simulink model "fusionAlg"  (R2018b)
settings: Solver=FixedStepDiscrete  StartTime=0.0  StopTime=inf  FixedStep=0.01  RelTol=1e-3
PostLoadFcn:
  | if any(exist('dsrtsu_mdlpostloadfcn', 'file') ~= 0), dsrtsu_mdlpostloadfcn('Execute', bdroot); end
model workspace (MAT data in the model file):
  handle : class17 (value not decoded)
(part 13 of 24)

== system fusionAlg/FUSION /FUS_DataAdapter/ARS308Adapter/leftFrontRadar/Subsystem1/OBJ_20 ==
  OBJ_01 : Inport
  Bus Creator : BusCreator  Inputs=2  OutDataTypeStr=Bus: FUS_UINT8_RESERVED_ST
      settings: InheritFromInputs=off
  Bus Creator1 : BusCreator  Inputs=17  OutDataTypeStr=Bus: FUS_RADAR_OBJ_ST  NonVirtualBus=on
      settings: InheritFromInputs=off
  Bus Selector1 : BusSelector  OutputSignals=RCS,VrelLat,VrelLong,DistLong,DistLat,ID,DynProp
  Constant{,1,8..10} (5 alike) : Constant  Value=0  OutDataTypeStr=uint8
  Constant{2..6} (5 alike) : Constant  Value=0  OutDataTypeStr=single
  Constant7 : Constant  OutDataTypeStr=uint8
  Data Type Conversion : DataTypeConversion  OutDataTypeStr=uint16
  Data Type Conversion1 : DataTypeConversion  OutDataTypeStr=uint8
  Switch : Switch  Criteria=u2 > Threshold  OutDataTypeStr=uint8
  <OBJ_01> : Outport
  wires:
  Constant1/1 -> Bus Creator/2
  Bus Creator1/1 -> <OBJ_01>/1
  Constant/1 -> Bus Creator/1
  OBJ_01/1 -> Bus Selector1/1
  Bus Creator/1 -> Bus Creator1/17
  Bus Selector1/1 -> Bus Creator1/1  "<RCS>"
  Constant2/1 -> Bus Creator1/2  "XPos_STD"
  Constant3/1 -> Bus Creator1/3  "YPos_STD"
  Constant4/1 -> Bus Creator1/4  "XVelRel_STD"
  Constant5/1 -> Bus Creator1/5  "XAccRel"
  Constant6/1 -> Bus Creator1/6  "ExstProb"
  Bus Selector1/2 -> Bus Creator1/7  "<VrelLat>"
  Bus Selector1/3 -> Bus Creator1/8  "<VrelLong>"
  Bus Selector1/4 -> Bus Creator1/9  "<DistLong>"
  Bus Selector1/5 -> Bus Creator1/10  "<DistLat>"
  Bus Selector1/6 -> Data Type Conversion/1  "<ID>"
  Data Type Conversion/1 -> Bus Creator1/11, Switch/2
  Constant8/1 -> Switch/3  "ValidFlag"
  Bus Selector1/7 -> Data Type Conversion1/1  "<DynProp>"
  Constant9/1 -> Bus Creator1/15  "Type"
  Constant10/1 -> Bus Creator1/16  "MeasFlag"
  Data Type Conversion1/1 -> Bus Creator1/14
  Constant7/1 -> Switch/1  "UpdateFlag"
  Switch/1 -> Bus Creator1/13, Bus Creator1/12

== system fusionAlg/FUSION /FUS_DataAdapter/ARS308Adapter/leftFrontRadar/Subsystem1/OBJ_21 ==
  OBJ_01 : Inport
  Bus Creator : BusCreator  Inputs=2  OutDataTypeStr=Bus: FUS_UINT8_RESERVED_ST
      settings: InheritFromInputs=off
  Bus Creator1 : BusCreator  Inputs=17  OutDataTypeStr=Bus: FUS_RADAR_OBJ_ST  NonVirtualBus=on
      settings: InheritFromInputs=off
  Bus Selector1 : BusSelector  OutputSignals=RCS,VrelLat,VrelLong,DistLong,DistLat,ID,DynProp
  Constant{,1,8..10} (5 alike) : Constant  Value=0  OutDataTypeStr=uint8
  Constant{2..6} (5 alike) : Constant  Value=0  OutDataTypeStr=single
  Constant7 : Constant  OutDataTypeStr=uint8
  Data Type Conversion : DataTypeConversion  OutDataTypeStr=uint16
  Data Type Conversion1 : DataTypeConversion  OutDataTypeStr=uint8
  Switch : Switch  Criteria=u2 > Threshold  OutDataTypeStr=uint8
  <OBJ_01> : Outport
  wires:
  Constant1/1 -> Bus Creator/2
  Bus Creator1/1 -> <OBJ_01>/1
  Constant/1 -> Bus Creator/1
  OBJ_01/1 -> Bus Selector1/1
  Bus Creator/1 -> Bus Creator1/17
  Bus Selector1/1 -> Bus Creator1/1  "<RCS>"
  Constant2/1 -> Bus Creator1/2  "XPos_STD"
  Constant3/1 -> Bus Creator1/3  "YPos_STD"
  Constant4/1 -> Bus Creator1/4  "XVelRel_STD"
  Constant5/1 -> Bus Creator1/5  "XAccRel"
  Constant6/1 -> Bus Creator1/6  "ExstProb"
  Bus Selector1/2 -> Bus Creator1/7  "<VrelLat>"
  Bus Selector1/3 -> Bus Creator1/8  "<VrelLong>"
  Bus Selector1/4 -> Bus Creator1/9  "<DistLong>"
  Bus Selector1/5 -> Bus Creator1/10  "<DistLat>"
  Bus Selector1/6 -> Data Type Conversion/1  "<ID>"
  Data Type Conversion/1 -> Bus Creator1/11, Switch/2
  Constant8/1 -> Switch/3  "ValidFlag"
  Bus Selector1/7 -> Data Type Conversion1/1  "<DynProp>"
  Constant9/1 -> Bus Creator1/15  "Type"
  Constant10/1 -> Bus Creator1/16  "MeasFlag"
  Data Type Conversion1/1 -> Bus Creator1/14
  Constant7/1 -> Switch/1  "UpdateFlag"
  Switch/1 -> Bus Creator1/13, Bus Creator1/12

== system fusionAlg/FUSION /FUS_DataAdapter/ARS308Adapter/leftFrontRadar/Subsystem1/OBJ_22 ==
  OBJ_01 : Inport
  Bus Creator : BusCreator  Inputs=2  OutDataTypeStr=Bus: FUS_UINT8_RESERVED_ST
      settings: InheritFromInputs=off
  Bus Creator1 : BusCreator  Inputs=17  OutDataTypeStr=Bus: FUS_RADAR_OBJ_ST  NonVirtualBus=on
      settings: InheritFromInputs=off
  Bus Selector1 : BusSelector  OutputSignals=RCS,VrelLat,VrelLong,DistLong,DistLat,ID,DynProp
  Constant{,1,8..10} (5 alike) : Constant  Value=0  OutDataTypeStr=uint8
  Constant{2..6} (5 alike) : Constant  Value=0  OutDataTypeStr=single
  Constant7 : Constant  OutDataTypeStr=uint8
  Data Type Conversion : DataTypeConversion  OutDataTypeStr=uint16
  Data Type Conversion1 : DataTypeConversion  OutDataTypeStr=uint8
  Switch : Switch  Criteria=u2 > Threshold  OutDataTypeStr=uint8
  <OBJ_01> : Outport
  wires:
  Constant1/1 -> Bus Creator/2
  Bus Creator1/1 -> <OBJ_01>/1
  Constant/1 -> Bus Creator/1
  OBJ_01/1 -> Bus Selector1/1
  Bus Creator/1 -> Bus Creator1/17
  Bus Selector1/1 -> Bus Creator1/1  "<RCS>"
  Constant2/1 -> Bus Creator1/2  "XPos_STD"
  Constant3/1 -> Bus Creator1/3  "YPos_STD"
  Constant4/1 -> Bus Creator1/4  "XVelRel_STD"
  Constant5/1 -> Bus Creator1/5  "XAccRel"
  Constant6/1 -> Bus Creator1/6  "ExstProb"
  Bus Selector1/2 -> Bus Creator1/7  "<VrelLat>"
  Bus Selector1/3 -> Bus Creator1/8  "<VrelLong>"
  Bus Selector1/4 -> Bus Creator1/9  "<DistLong>"
  Bus Selector1/5 -> Bus Creator1/10  "<DistLat>"
  Bus Selector1/6 -> Data Type Conversion/1  "<ID>"
  Data Type Conversion/1 -> Bus Creator1/11, Switch/2
  Constant8/1 -> Switch/3  "ValidFlag"
  Bus Selector1/7 -> Data Type Conversion1/1  "<DynProp>"
  Constant9/1 -> Bus Creator1/15  "Type"
  Constant10/1 -> Bus Creator1/16  "MeasFlag"
  Data Type Conversion1/1 -> Bus Creator1/14
  Constant7/1 -> Switch/1  "UpdateFlag"
  Switch/1 -> Bus Creator1/13, Bus Creator1/12

== system fusionAlg/FUSION /FUS_DataAdapter/ARS308Adapter/leftFrontRadar/Subsystem1/OBJ_23 ==
  OBJ_01 : Inport
  Bus Creator : BusCreator  Inputs=2  OutDataTypeStr=Bus: FUS_UINT8_RESERVED_ST
      settings: InheritFromInputs=off
  Bus Creator1 : BusCreator  Inputs=17  OutDataTypeStr=Bus: FUS_RADAR_OBJ_ST  NonVirtualBus=on
      settings: InheritFromInputs=off
  Bus Selector1 : BusSelector  OutputSignals=RCS,VrelLat,VrelLong,DistLong,DistLat,ID,DynProp
  Constant{,1,8..10} (5 alike) : Constant  Value=0  OutDataTypeStr=uint8
  Constant{2..6} (5 alike) : Constant  Value=0  OutDataTypeStr=single
  Constant7 : Constant  OutDataTypeStr=uint8
  Data Type Conversion : DataTypeConversion  OutDataTypeStr=uint16
  Data Type Conversion1 : DataTypeConversion  OutDataTypeStr=uint8
  Switch : Switch  Criteria=u2 > Threshold  OutDataTypeStr=uint8
  <OBJ_01> : Outport
  wires:
  Constant1/1 -> Bus Creator/2
  Bus Creator1/1 -> <OBJ_01>/1
  Constant/1 -> Bus Creator/1
  OBJ_01/1 -> Bus Selector1/1
  Bus Creator/1 -> Bus Creator1/17
  Bus Selector1/1 -> Bus Creator1/1  "<RCS>"
  Constant2/1 -> Bus Creator1/2  "XPos_STD"
  Constant3/1 -> Bus Creator1/3  "YPos_STD"
  Constant4/1 -> Bus Creator1/4  "XVelRel_STD"
  Constant5/1 -> Bus Creator1/5  "XAccRel"
  Constant6/1 -> Bus Creator1/6  "ExstProb"
  Bus Selector1/2 -> Bus Creator1/7  "<VrelLat>"
  Bus Selector1/3 -> Bus Creator1/8  "<VrelLong>"
  Bus Selector1/4 -> Bus Creator1/9  "<DistLong>"
  Bus Selector1/5 -> Bus Creator1/10  "<DistLat>"
  Bus Selector1/6 -> Data Type Conversion/1  "<ID>"
  Data Type Conversion/1 -> Bus Creator1/11, Switch/2
  Constant8/1 -> Switch/3  "ValidFlag"
  Bus Selector1/7 -> Data Type Conversion1/1  "<DynProp>"
  Constant9/1 -> Bus Creator1/15  "Type"
  Constant10/1 -> Bus Creator1/16  "MeasFlag"
  Data Type Conversion1/1 -> Bus Creator1/14
  Constant7/1 -> Switch/1  "UpdateFlag"
  Switch/1 -> Bus Creator1/13, Bus Creator1/12

== system fusionAlg/FUSION /FUS_DataAdapter/ARS308Adapter/leftFrontRadar/Subsystem1/OBJ_24 ==
  OBJ_01 : Inport
  Bus Creator : BusCreator  Inputs=2  OutDataTypeStr=Bus: FUS_UINT8_RESERVED_ST
      settings: InheritFromInputs=off
  Bus Creator1 : BusCreator  Inputs=17  OutDataTypeStr=Bus: FUS_RADAR_OBJ_ST  NonVirtualBus=on
      settings: InheritFromInputs=off
  Bus Selector1 : BusSelector  OutputSignals=RCS,VrelLat,VrelLong,DistLong,DistLat,ID,DynProp
  Constant{,1,8..10} (5 alike) : Constant  Value=0  OutDataTypeStr=uint8
  Constant{2..6} (5 alike) : Constant  Value=0  OutDataTypeStr=single
  Constant7 : Constant  OutDataTypeStr=uint8
  Data Type Conversion : DataTypeConversion  OutDataTypeStr=uint16
  Data Type Conversion1 : DataTypeConversion  OutDataTypeStr=uint8
  Switch : Switch  Criteria=u2 > Threshold  OutDataTypeStr=uint8
  <OBJ_01> : Outport
  wires:
  Constant1/1 -> Bus Creator/2
  Bus Creator1/1 -> <OBJ_01>/1
  Constant/1 -> Bus Creator/1
  OBJ_01/1 -> Bus Selector1/1
  Bus Creator/1 -> Bus Creator1/17
  Bus Selector1/1 -> Bus Creator1/1  "<RCS>"
  Constant2/1 -> Bus Creator1/2  "XPos_STD"
  Constant3/1 -> Bus Creator1/3  "YPos_STD"
  Constant4/1 -> Bus Creator1/4  "XVelRel_STD"
  Constant5/1 -> Bus Creator1/5  "XAccRel"
  Constant6/1 -> Bus Creator1/6  "ExstProb"
  Bus Selector1/2 -> Bus Creator1/7  "<VrelLat>"
  Bus Selector1/3 -> Bus Creator1/8  "<VrelLong>"
  Bus Selector1/4 -> Bus Creator1/9  "<DistLong>"
  Bus Selector1/5 -> Bus Creator1/10  "<DistLat>"
  Bus Selector1/6 -> Data Type Conversion/1  "<ID>"
  Data Type Conversion/1 -> Bus Creator1/11, Switch/2
  Constant8/1 -> Switch/3  "ValidFlag"
  Bus Selector1/7 -> Data Type Conversion1/1  "<DynProp>"
  Constant9/1 -> Bus Creator1/15  "Type"
  Constant10/1 -> Bus Creator1/16  "MeasFlag"
  Data Type Conversion1/1 -> Bus Creator1/14
  Constant7/1 -> Switch/1  "UpdateFlag"
  Switch/1 -> Bus Creator1/13, Bus Creator1/12

== system fusionAlg/FUSION /FUS_DataAdapter/ARS308Adapter/leftFrontRadar/Subsystem1/OBJ_25 ==
  OBJ_01 : Inport
  Bus Creator : BusCreator  Inputs=2  OutDataTypeStr=Bus: FUS_UINT8_RESERVED_ST
      settings: InheritFromInputs=off
  Bus Creator1 : BusCreator  Inputs=17  OutDataTypeStr=Bus: FUS_RADAR_OBJ_ST  NonVirtualBus=on
      settings: InheritFromInputs=off
  Bus Selector1 : BusSelector  OutputSignals=RCS,VrelLat,VrelLong,DistLong,DistLat,ID,DynProp
  Constant{,1,8..10} (5 alike) : Constant  Value=0  OutDataTypeStr=uint8
  Constant{2..6} (5 alike) : Constant  Value=0  OutDataTypeStr=single
  Constant7 : Constant  OutDataTypeStr=uint8
  Data Type Conversion : DataTypeConversion  OutDataTypeStr=uint16
  Data Type Conversion1 : DataTypeConversion  OutDataTypeStr=uint8
  Switch : Switch  Criteria=u2 > Threshold  OutDataTypeStr=uint8
  <OBJ_01> : Outport
  wires:
  Constant1/1 -> Bus Creator/2
  Bus Creator1/1 -> <OBJ_01>/1
  Constant/1 -> Bus Creator/1
  OBJ_01/1 -> Bus Selector1/1
  Bus Creator/1 -> Bus Creator1/17
  Bus Selector1/1 -> Bus Creator1/1  "<RCS>"
  Constant2/1 -> Bus Creator1/2  "XPos_STD"
  Constant3/1 -> Bus Creator1/3  "YPos_STD"
  Constant4/1 -> Bus Creator1/4  "XVelRel_STD"
  Constant5/1 -> Bus Creator1/5  "XAccRel"
  Constant6/1 -> Bus Creator1/6  "ExstProb"
  Bus Selector1/2 -> Bus Creator1/7  "<VrelLat>"
  Bus Selector1/3 -> Bus Creator1/8  "<VrelLong>"
  Bus Selector1/4 -> Bus Creator1/9  "<DistLong>"
  Bus Selector1/5 -> Bus Creator1/10  "<DistLat>"
  Bus Selector1/6 -> Data Type Conversion/1  "<ID>"
  Data Type Conversion/1 -> Bus Creator1/11, Switch/2
  Constant8/1 -> Switch/3  "ValidFlag"
  Bus Selector1/7 -> Data Type Conversion1/1  "<DynProp>"
  Constant9/1 -> Bus Creator1/15  "Type"
  Constant10/1 -> Bus Creator1/16  "MeasFlag"
  Data Type Conversion1/1 -> Bus Creator1/14
  Constant7/1 -> Switch/1  "UpdateFlag"
  Switch/1 -> Bus Creator1/13, Bus Creator1/12

== system fusionAlg/FUSION /FUS_DataAdapter/ARS308Adapter/leftFrontRadar/Subsystem1/OBJ_26 ==
  OBJ_01 : Inport
  Bus Creator : BusCreator  Inputs=2  OutDataTypeStr=Bus: FUS_UINT8_RESERVED_ST
      settings: InheritFromInputs=off
  Bus Creator1 : BusCreator  Inputs=17  OutDataTypeStr=Bus: FUS_RADAR_OBJ_ST  NonVirtualBus=on
      settings: InheritFromInputs=off
  Bus Selector1 : BusSelector  OutputSignals=RCS,VrelLat,VrelLong,DistLong,DistLat,ID,DynProp
  Constant{,1,8..10} (5 alike) : Constant  Value=0  OutDataTypeStr=uint8
  Constant{2..6} (5 alike) : Constant  Value=0  OutDataTypeStr=single
  Constant7 : Constant  OutDataTypeStr=uint8
  Data Type Conversion : DataTypeConversion  OutDataTypeStr=uint16
  Data Type Conversion1 : DataTypeConversion  OutDataTypeStr=uint8
  Switch : Switch  Criteria=u2 > Threshold  OutDataTypeStr=uint8
  <OBJ_01> : Outport
  wires:
  Constant1/1 -> Bus Creator/2
  Bus Creator1/1 -> <OBJ_01>/1
  Constant/1 -> Bus Creator/1
  OBJ_01/1 -> Bus Selector1/1
  Bus Creator/1 -> Bus Creator1/17
  Bus Selector1/1 -> Bus Creator1/1  "<RCS>"
  Constant2/1 -> Bus Creator1/2  "XPos_STD"
  Constant3/1 -> Bus Creator1/3  "YPos_STD"
  Constant4/1 -> Bus Creator1/4  "XVelRel_STD"
  Constant5/1 -> Bus Creator1/5  "XAccRel"
  Constant6/1 -> Bus Creator1/6  "ExstProb"
  Bus Selector1/2 -> Bus Creator1/7  "<VrelLat>"
  Bus Selector1/3 -> Bus Creator1/8  "<VrelLong>"
  Bus Selector1/4 -> Bus Creator1/9  "<DistLong>"
  Bus Selector1/5 -> Bus Creator1/10  "<DistLat>"
  Bus Selector1/6 -> Data Type Conversion/1  "<ID>"
  Data Type Conversion/1 -> Bus Creator1/11, Switch/2
  Constant8/1 -> Switch/3  "ValidFlag"
  Bus Selector1/7 -> Data Type Conversion1/1  "<DynProp>"
  Constant9/1 -> Bus Creator1/15  "Type"
  Constant10/1 -> Bus Creator1/16  "MeasFlag"
  Data Type Conversion1/1 -> Bus Creator1/14
  Constant7/1 -> Switch/1  "UpdateFlag"
  Switch/1 -> Bus Creator1/13, Bus Creator1/12

== system fusionAlg/FUSION /FUS_DataAdapter/ARS308Adapter/leftFrontRadar/Subsystem1/OBJ_27 ==
  OBJ_01 : Inport
  Bus Creator : BusCreator  Inputs=2  OutDataTypeStr=Bus: FUS_UINT8_RESERVED_ST
      settings: InheritFromInputs=off
  Bus Creator1 : BusCreator  Inputs=17  OutDataTypeStr=Bus: FUS_RADAR_OBJ_ST  NonVirtualBus=on
      settings: InheritFromInputs=off
  Bus Selector1 : BusSelector  OutputSignals=RCS,VrelLat,VrelLong,DistLong,DistLat,ID,DynProp
  Constant{,1,8..10} (5 alike) : Constant  Value=0  OutDataTypeStr=uint8
  Constant{2..6} (5 alike) : Constant  Value=0  OutDataTypeStr=single
  Constant7 : Constant  OutDataTypeStr=uint8
  Data Type Conversion : DataTypeConversion  OutDataTypeStr=uint16
  Data Type Conversion1 : DataTypeConversion  OutDataTypeStr=uint8
  Switch : Switch  Criteria=u2 > Threshold  OutDataTypeStr=uint8
  <OBJ_01> : Outport
  wires:
  Constant1/1 -> Bus Creator/2
  Bus Creator1/1 -> <OBJ_01>/1
  Constant/1 -> Bus Creator/1
  OBJ_01/1 -> Bus Selector1/1
  Bus Creator/1 -> Bus Creator1/17
  Bus Selector1/1 -> Bus Creator1/1  "<RCS>"
  Constant2/1 -> Bus Creator1/2  "XPos_STD"
  Constant3/1 -> Bus Creator1/3  "YPos_STD"
  Constant4/1 -> Bus Creator1/4  "XVelRel_STD"
  Constant5/1 -> Bus Creator1/5  "XAccRel"
  Constant6/1 -> Bus Creator1/6  "ExstProb"
  Bus Selector1/2 -> Bus Creator1/7  "<VrelLat>"
  Bus Selector1/3 -> Bus Creator1/8  "<VrelLong>"
  Bus Selector1/4 -> Bus Creator1/9  "<DistLong>"
  Bus Selector1/5 -> Bus Creator1/10  "<DistLat>"
  Bus Selector1/6 -> Data Type Conversion/1  "<ID>"
  Data Type Conversion/1 -> Bus Creator1/11, Switch/2
  Constant8/1 -> Switch/3  "ValidFlag"
  Bus Selector1/7 -> Data Type Conversion1/1  "<DynProp>"
  Constant9/1 -> Bus Creator1/15  "Type"
  Constant10/1 -> Bus Creator1/16  "MeasFlag"
  Data Type Conversion1/1 -> Bus Creator1/14
  Constant7/1 -> Switch/1  "UpdateFlag"
  Switch/1 -> Bus Creator1/13, Bus Creator1/12

== system fusionAlg/FUSION /FUS_DataAdapter/ARS308Adapter/leftFrontRadar/Subsystem1/OBJ_28 ==
  OBJ_01 : Inport
  Bus Creator : BusCreator  Inputs=2  OutDataTypeStr=Bus: FUS_UINT8_RESERVED_ST
      settings: InheritFromInputs=off
  Bus Creator1 : BusCreator  Inputs=17  OutDataTypeStr=Bus: FUS_RADAR_OBJ_ST  NonVirtualBus=on
      settings: InheritFromInputs=off
  Bus Selector1 : BusSelector  OutputSignals=RCS,VrelLat,VrelLong,DistLong,DistLat,ID,DynProp
  Constant{,1,8..10} (5 alike) : Constant  Value=0  OutDataTypeStr=uint8
  Constant{2..6} (5 alike) : Constant  Value=0  OutDataTypeStr=single
  Constant7 : Constant  OutDataTypeStr=uint8
  Data Type Conversion : DataTypeConversion  OutDataTypeStr=uint16
  Data Type Conversion1 : DataTypeConversion  OutDataTypeStr=uint8
  Switch : Switch  Criteria=u2 > Threshold  OutDataTypeStr=uint8
  <OBJ_01> : Outport
  wires:
  Constant1/1 -> Bus Creator/2
  Bus Creator1/1 -> <OBJ_01>/1
  Constant/1 -> Bus Creator/1
  OBJ_01/1 -> Bus Selector1/1
  Bus Creator/1 -> Bus Creator1/17
  Bus Selector1/1 -> Bus Creator1/1  "<RCS>"
  Constant2/1 -> Bus Creator1/2  "XPos_STD"
  Constant3/1 -> Bus Creator1/3  "YPos_STD"
  Constant4/1 -> Bus Creator1/4  "XVelRel_STD"
  Constant5/1 -> Bus Creator1/5  "XAccRel"
  Constant6/1 -> Bus Creator1/6  "ExstProb"
  Bus Selector1/2 -> Bus Creator1/7  "<VrelLat>"
  Bus Selector1/3 -> Bus Creator1/8  "<VrelLong>"
  Bus Selector1/4 -> Bus Creator1/9  "<DistLong>"
  Bus Selector1/5 -> Bus Creator1/10  "<DistLat>"
  Bus Selector1/6 -> Data Type Conversion/1  "<ID>"
  Data Type Conversion/1 -> Bus Creator1/11, Switch/2
  Constant8/1 -> Switch/3  "ValidFlag"
  Bus Selector1/7 -> Data Type Conversion1/1  "<DynProp>"
  Constant9/1 -> Bus Creator1/15  "Type"
  Constant10/1 -> Bus Creator1/16  "MeasFlag"
  Data Type Conversion1/1 -> Bus Creator1/14
  Constant7/1 -> Switch/1  "UpdateFlag"
  Switch/1 -> Bus Creator1/13, Bus Creator1/12

== system fusionAlg/FUSION /FUS_DataAdapter/ARS308Adapter/leftFrontRadar/Subsystem1/OBJ_29 ==
  OBJ_01 : Inport
  Bus Creator : BusCreator  Inputs=2  OutDataTypeStr=Bus: FUS_UINT8_RESERVED_ST
      settings: InheritFromInputs=off
  Bus Creator1 : BusCreator  Inputs=17  OutDataTypeStr=Bus: FUS_RADAR_OBJ_ST  NonVirtualBus=on
      settings: InheritFromInputs=off
  Bus Selector1 : BusSelector  OutputSignals=RCS,VrelLat,VrelLong,DistLong,DistLat,ID,DynProp
  Constant{,1,8..10} (5 alike) : Constant  Value=0  OutDataTypeStr=uint8
  Constant{2..6} (5 alike) : Constant  Value=0  OutDataTypeStr=single
  Constant7 : Constant  OutDataTypeStr=uint8
  Data Type Conversion : DataTypeConversion  OutDataTypeStr=uint16
  Data Type Conversion1 : DataTypeConversion  OutDataTypeStr=uint8
  Switch : Switch  Criteria=u2 > Threshold  OutDataTypeStr=uint8
  <OBJ_01> : Outport
  wires:
  Constant1/1 -> Bus Creator/2
  Bus Creator1/1 -> <OBJ_01>/1
  Constant/1 -> Bus Creator/1
  OBJ_01/1 -> Bus Selector1/1
  Bus Creator/1 -> Bus Creator1/17
  Bus Selector1/1 -> Bus Creator1/1  "<RCS>"
  Constant2/1 -> Bus Creator1/2  "XPos_STD"
  Constant3/1 -> Bus Creator1/3  "YPos_STD"
  Constant4/1 -> Bus Creator1/4  "XVelRel_STD"
  Constant5/1 -> Bus Creator1/5  "XAccRel"
  Constant6/1 -> Bus Creator1/6  "ExstProb"
  Bus Selector1/2 -> Bus Creator1/7  "<VrelLat>"
  Bus Selector1/3 -> Bus Creator1/8  "<VrelLong>"
  Bus Selector1/4 -> Bus Creator1/9  "<DistLong>"
  Bus Selector1/5 -> Bus Creator1/10  "<DistLat>"
  Bus Selector1/6 -> Data Type Conversion/1  "<ID>"
  Data Type Conversion/1 -> Bus Creator1/11, Switch/2
  Constant8/1 -> Switch/3  "ValidFlag"
  Bus Selector1/7 -> Data Type Conversion1/1  "<DynProp>"
  Constant9/1 -> Bus Creator1/15  "Type"
  Constant10/1 -> Bus Creator1/16  "MeasFlag"
  Data Type Conversion1/1 -> Bus Creator1/14
  Constant7/1 -> Switch/1  "UpdateFlag"
  Switch/1 -> Bus Creator1/13, Bus Creator1/12

== system fusionAlg/FUSION /FUS_DataAdapter/ARS308Adapter/leftFrontRadar/Subsystem1/OBJ_3 ==
  OBJ_01 : Inport
  Bus Creator : BusCreator  Inputs=2  OutDataTypeStr=Bus: FUS_UINT8_RESERVED_ST
      settings: InheritFromInputs=off
  Bus Creator1 : BusCreator  Inputs=17  OutDataTypeStr=Bus: FUS_RADAR_OBJ_ST  NonVirtualBus=on
      settings: InheritFromInputs=off
  Bus Selector1 : BusSelector  OutputSignals=RCS,VrelLat,VrelLong,DistLong,DistLat,ID,DynProp
  Constant{,1,8..10} (5 alike) : Constant  Value=0  OutDataTypeStr=uint8
  Constant{2..6} (5 alike) : Constant  Value=0  OutDataTypeStr=single
  Constant7 : Constant  OutDataTypeStr=uint8
  Data Type Conversion : DataTypeConversion  OutDataTypeStr=uint16
  Data Type Conversion1 : DataTypeConversion  OutDataTypeStr=uint8
  Switch : Switch  Criteria=u2 > Threshold  OutDataTypeStr=uint8
  <OBJ_01> : Outport
  wires:
  Constant1/1 -> Bus Creator/2
  Bus Creator1/1 -> <OBJ_01>/1
  Constant/1 -> Bus Creator/1
  OBJ_01/1 -> Bus Selector1/1
  Bus Creator/1 -> Bus Creator1/17
  Bus Selector1/1 -> Bus Creator1/1  "<RCS>"
  Constant2/1 -> Bus Creator1/2  "XPos_STD"
  Constant3/1 -> Bus Creator1/3  "YPos_STD"
  Constant4/1 -> Bus Creator1/4  "XVelRel_STD"
  Constant5/1 -> Bus Creator1/5  "XAccRel"
  Constant6/1 -> Bus Creator1/6  "ExstProb"
  Bus Selector1/2 -> Bus Creator1/7  "<VrelLat>"
  Bus Selector1/3 -> Bus Creator1/8  "<VrelLong>"
  Bus Selector1/4 -> Bus Creator1/9  "<DistLong>"
  Bus Selector1/5 -> Bus Creator1/10  "<DistLat>"
  Bus Selector1/6 -> Data Type Conversion/1  "<ID>"
  Data Type Conversion/1 -> Bus Creator1/11, Switch/2
  Constant8/1 -> Switch/3  "ValidFlag"
  Bus Selector1/7 -> Data Type Conversion1/1  "<DynProp>"
  Constant9/1 -> Bus Creator1/15  "Type"
  Constant10/1 -> Bus Creator1/16  "MeasFlag"
  Data Type Conversion1/1 -> Bus Creator1/14
  Constant7/1 -> Switch/1  "UpdateFlag"
  Switch/1 -> Bus Creator1/13, Bus Creator1/12

== system fusionAlg/FUSION /FUS_DataAdapter/ARS308Adapter/leftFrontRadar/Subsystem1/OBJ_30 ==
  OBJ_01 : Inport
  Bus Creator : BusCreator  Inputs=2  OutDataTypeStr=Bus: FUS_UINT8_RESERVED_ST
      settings: InheritFromInputs=off
  Bus Creator1 : BusCreator  Inputs=17  OutDataTypeStr=Bus: FUS_RADAR_OBJ_ST  NonVirtualBus=on
      settings: InheritFromInputs=off
  Bus Selector1 : BusSelector  OutputSignals=RCS,VrelLat,VrelLong,DistLong,DistLat,ID,DynProp
  Constant{,1,8..10} (5 alike) : Constant  Value=0  OutDataTypeStr=uint8
  Constant{2..6} (5 alike) : Constant  Value=0  OutDataTypeStr=single
  Constant7 : Constant  OutDataTypeStr=uint8
  Data Type Conversion : DataTypeConversion  OutDataTypeStr=uint16
  Data Type Conversion1 : DataTypeConversion  OutDataTypeStr=uint8
  Switch : Switch  Criteria=u2 > Threshold  OutDataTypeStr=uint8
  <OBJ_01> : Outport
  wires:
  Constant1/1 -> Bus Creator/2
  Bus Creator1/1 -> <OBJ_01>/1
  Constant/1 -> Bus Creator/1
  OBJ_01/1 -> Bus Selector1/1
  Bus Creator/1 -> Bus Creator1/17
  Bus Selector1/1 -> Bus Creator1/1  "<RCS>"
  Constant2/1 -> Bus Creator1/2  "XPos_STD"
  Constant3/1 -> Bus Creator1/3  "YPos_STD"
  Constant4/1 -> Bus Creator1/4  "XVelRel_STD"
  Constant5/1 -> Bus Creator1/5  "XAccRel"
  Constant6/1 -> Bus Creator1/6  "ExstProb"
  Bus Selector1/2 -> Bus Creator1/7  "<VrelLat>"
  Bus Selector1/3 -> Bus Creator1/8  "<VrelLong>"
  Bus Selector1/4 -> Bus Creator1/9  "<DistLong>"
  Bus Selector1/5 -> Bus Creator1/10  "<DistLat>"
  Bus Selector1/6 -> Data Type Conversion/1  "<ID>"
  Data Type Conversion/1 -> Bus Creator1/11, Switch/2
  Constant8/1 -> Switch/3  "ValidFlag"
  Bus Selector1/7 -> Data Type Conversion1/1  "<DynProp>"
  Constant9/1 -> Bus Creator1/15  "Type"
  Constant10/1 -> Bus Creator1/16  "MeasFlag"
  Data Type Conversion1/1 -> Bus Creator1/14
  Constant7/1 -> Switch/1  "UpdateFlag"
  Switch/1 -> Bus Creator1/13, Bus Creator1/12

== system fusionAlg/FUSION /FUS_DataAdapter/ARS308Adapter/leftFrontRadar/Subsystem1/OBJ_31 ==
  OBJ_01 : Inport
  Bus Creator : BusCreator  Inputs=2  OutDataTypeStr=Bus: FUS_UINT8_RESERVED_ST
      settings: InheritFromInputs=off
  Bus Creator1 : BusCreator  Inputs=17  OutDataTypeStr=Bus: FUS_RADAR_OBJ_ST  NonVirtualBus=on
      settings: InheritFromInputs=off
  Bus Selector1 : BusSelector  OutputSignals=RCS,VrelLat,VrelLong,DistLong,DistLat,ID,DynProp
  Constant{,1,8..10} (5 alike) : Constant  Value=0  OutDataTypeStr=uint8
  Constant{2..6} (5 alike) : Constant  Value=0  OutDataTypeStr=single
  Constant7 : Constant  OutDataTypeStr=uint8
  Data Type Conversion : DataTypeConversion  OutDataTypeStr=uint16
  Data Type Conversion1 : DataTypeConversion  OutDataTypeStr=uint8
  Switch : Switch  Criteria=u2 > Threshold  OutDataTypeStr=uint8
  <OBJ_01> : Outport
  wires:
  Constant1/1 -> Bus Creator/2
  Bus Creator1/1 -> <OBJ_01>/1
  Constant/1 -> Bus Creator/1
  OBJ_01/1 -> Bus Selector1/1
  Bus Creator/1 -> Bus Creator1/17
  Bus Selector1/1 -> Bus Creator1/1  "<RCS>"
  Constant2/1 -> Bus Creator1/2  "XPos_STD"
  Constant3/1 -> Bus Creator1/3  "YPos_STD"
  Constant4/1 -> Bus Creator1/4  "XVelRel_STD"
  Constant5/1 -> Bus Creator1/5  "XAccRel"
  Constant6/1 -> Bus Creator1/6  "ExstProb"
  Bus Selector1/2 -> Bus Creator1/7  "<VrelLat>"
  Bus Selector1/3 -> Bus Creator1/8  "<VrelLong>"
  Bus Selector1/4 -> Bus Creator1/9  "<DistLong>"
  Bus Selector1/5 -> Bus Creator1/10  "<DistLat>"
  Bus Selector1/6 -> Data Type Conversion/1  "<ID>"
  Data Type Conversion/1 -> Bus Creator1/11, Switch/2
  Constant8/1 -> Switch/3  "ValidFlag"
  Bus Selector1/7 -> Data Type Conversion1/1  "<DynProp>"
  Constant9/1 -> Bus Creator1/15  "Type"
  Constant10/1 -> Bus Creator1/16  "MeasFlag"
  Data Type Conversion1/1 -> Bus Creator1/14
  Constant7/1 -> Switch/1  "UpdateFlag"
  Switch/1 -> Bus Creator1/13, Bus Creator1/12

== system fusionAlg/FUSION /FUS_DataAdapter/ARS308Adapter/leftFrontRadar/Subsystem1/OBJ_32 ==
  OBJ_01 : Inport
  Bus Creator : BusCreator  Inputs=2  OutDataTypeStr=Bus: FUS_UINT8_RESERVED_ST
      settings: InheritFromInputs=off
  Bus Creator1 : BusCreator  Inputs=17  OutDataTypeStr=Bus: FUS_RADAR_OBJ_ST  NonVirtualBus=on
      settings: InheritFromInputs=off
  Bus Selector1 : BusSelector  OutputSignals=RCS,VrelLat,VrelLong,DistLong,DistLat,ID,DynProp
  Constant{,1,8..10} (5 alike) : Constant  Value=0  OutDataTypeStr=uint8
  Constant{2..6} (5 alike) : Constant  Value=0  OutDataTypeStr=single
  Constant7 : Constant  OutDataTypeStr=uint8
  Data Type Conversion : DataTypeConversion  OutDataTypeStr=uint16
  Data Type Conversion1 : DataTypeConversion  OutDataTypeStr=uint8
  Switch : Switch  Criteria=u2 > Threshold  OutDataTypeStr=uint8
  <OBJ_01> : Outport
  wires:
  Constant1/1 -> Bus Creator/2
  Bus Creator1/1 -> <OBJ_01>/1
  Constant/1 -> Bus Creator/1
  OBJ_01/1 -> Bus Selector1/1
  Bus Creator/1 -> Bus Creator1/17
  Bus Selector1/1 -> Bus Creator1/1  "<RCS>"
  Constant2/1 -> Bus Creator1/2  "XPos_STD"
  Constant3/1 -> Bus Creator1/3  "YPos_STD"
  Constant4/1 -> Bus Creator1/4  "XVelRel_STD"
  Constant5/1 -> Bus Creator1/5  "XAccRel"
  Constant6/1 -> Bus Creator1/6  "ExstProb"
  Bus Selector1/2 -> Bus Creator1/7  "<VrelLat>"
  Bus Selector1/3 -> Bus Creator1/8  "<VrelLong>"
  Bus Selector1/4 -> Bus Creator1/9  "<DistLong>"
  Bus Selector1/5 -> Bus Creator1/10  "<DistLat>"
  Bus Selector1/6 -> Data Type Conversion/1  "<ID>"
  Data Type Conversion/1 -> Bus Creator1/11, Switch/2
  Constant8/1 -> Switch/3  "ValidFlag"
  Bus Selector1/7 -> Data Type Conversion1/1  "<DynProp>"
  Constant9/1 -> Bus Creator1/15  "Type"
  Constant10/1 -> Bus Creator1/16  "MeasFlag"
  Data Type Conversion1/1 -> Bus Creator1/14
  Constant7/1 -> Switch/1  "UpdateFlag"
  Switch/1 -> Bus Creator1/13, Bus Creator1/12

== system fusionAlg/FUSION /FUS_DataAdapter/ARS308Adapter/leftFrontRadar/Subsystem1/OBJ_33 ==
  OBJ_01 : Inport
  Bus Creator : BusCreator  Inputs=2  OutDataTypeStr=Bus: FUS_UINT8_RESERVED_ST
      settings: InheritFromInputs=off
  Bus Creator1 : BusCreator  Inputs=17  OutDataTypeStr=Bus: FUS_RADAR_OBJ_ST  NonVirtualBus=on
      settings: InheritFromInputs=off
  Bus Selector1 : BusSelector  OutputSignals=RCS,VrelLat,VrelLong,DistLong,DistLat,ID,DynProp
  Constant{,1,8..10} (5 alike) : Constant  Value=0  OutDataTypeStr=uint8
  Constant{2..6} (5 alike) : Constant  Value=0  OutDataTypeStr=single
  Constant7 : Constant  OutDataTypeStr=uint8
  Data Type Conversion : DataTypeConversion  OutDataTypeStr=uint16
  Data Type Conversion1 : DataTypeConversion  OutDataTypeStr=uint8
  Switch : Switch  Criteria=u2 > Threshold  OutDataTypeStr=uint8
  <OBJ_01> : Outport
  wires:
  Constant1/1 -> Bus Creator/2
  Bus Creator1/1 -> <OBJ_01>/1
  Constant/1 -> Bus Creator/1
  OBJ_01/1 -> Bus Selector1/1
  Bus Creator/1 -> Bus Creator1/17
  Bus Selector1/1 -> Bus Creator1/1  "<RCS>"
  Constant2/1 -> Bus Creator1/2  "XPos_STD"
  Constant3/1 -> Bus Creator1/3  "YPos_STD"
  Constant4/1 -> Bus Creator1/4  "XVelRel_STD"
  Constant5/1 -> Bus Creator1/5  "XAccRel"
  Constant6/1 -> Bus Creator1/6  "ExstProb"
  Bus Selector1/2 -> Bus Creator1/7  "<VrelLat>"
  Bus Selector1/3 -> Bus Creator1/8  "<VrelLong>"
  Bus Selector1/4 -> Bus Creator1/9  "<DistLong>"
  Bus Selector1/5 -> Bus Creator1/10  "<DistLat>"
  Bus Selector1/6 -> Data Type Conversion/1  "<ID>"
  Data Type Conversion/1 -> Bus Creator1/11, Switch/2
  Constant8/1 -> Switch/3  "ValidFlag"
  Bus Selector1/7 -> Data Type Conversion1/1  "<DynProp>"
  Constant9/1 -> Bus Creator1/15  "Type"
  Constant10/1 -> Bus Creator1/16  "MeasFlag"
  Data Type Conversion1/1 -> Bus Creator1/14
  Constant7/1 -> Switch/1  "UpdateFlag"
  Switch/1 -> Bus Creator1/13, Bus Creator1/12

== system fusionAlg/FUSION /FUS_DataAdapter/ARS308Adapter/leftFrontRadar/Subsystem1/OBJ_34 ==
  OBJ_01 : Inport
  Bus Creator : BusCreator  Inputs=2  OutDataTypeStr=Bus: FUS_UINT8_RESERVED_ST
      settings: InheritFromInputs=off
  Bus Creator1 : BusCreator  Inputs=17  OutDataTypeStr=Bus: FUS_RADAR_OBJ_ST  NonVirtualBus=on
      settings: InheritFromInputs=off
  Bus Selector1 : BusSelector  OutputSignals=RCS,VrelLat,VrelLong,DistLong,DistLat,ID,DynProp
  Constant{,1,8..10} (5 alike) : Constant  Value=0  OutDataTypeStr=uint8
  Constant{2..6} (5 alike) : Constant  Value=0  OutDataTypeStr=single
  Constant7 : Constant  OutDataTypeStr=uint8
  Data Type Conversion : DataTypeConversion  OutDataTypeStr=uint16
  Data Type Conversion1 : DataTypeConversion  OutDataTypeStr=uint8
  Switch : Switch  Criteria=u2 > Threshold  OutDataTypeStr=uint8
  <OBJ_01> : Outport
  wires:
  Constant1/1 -> Bus Creator/2
  Bus Creator1/1 -> <OBJ_01>/1
  Constant/1 -> Bus Creator/1
  OBJ_01/1 -> Bus Selector1/1
  Bus Creator/1 -> Bus Creator1/17
  Bus Selector1/1 -> Bus Creator1/1  "<RCS>"
  Constant2/1 -> Bus Creator1/2  "XPos_STD"
  Constant3/1 -> Bus Creator1/3  "YPos_STD"
  Constant4/1 -> Bus Creator1/4  "XVelRel_STD"
  Constant5/1 -> Bus Creator1/5  "XAccRel"
  Constant6/1 -> Bus Creator1/6  "ExstProb"
  Bus Selector1/2 -> Bus Creator1/7  "<VrelLat>"
  Bus Selector1/3 -> Bus Creator1/8  "<VrelLong>"
  Bus Selector1/4 -> Bus Creator1/9  "<DistLong>"
  Bus Selector1/5 -> Bus Creator1/10  "<DistLat>"
  Bus Selector1/6 -> Data Type Conversion/1  "<ID>"
  Data Type Conversion/1 -> Bus Creator1/11, Switch/2
  Constant8/1 -> Switch/3  "ValidFlag"
  Bus Selector1/7 -> Data Type Conversion1/1  "<DynProp>"
  Constant9/1 -> Bus Creator1/15  "Type"
  Constant10/1 -> Bus Creator1/16  "MeasFlag"
  Data Type Conversion1/1 -> Bus Creator1/14
  Constant7/1 -> Switch/1  "UpdateFlag"
  Switch/1 -> Bus Creator1/13, Bus Creator1/12

== system fusionAlg/FUSION /FUS_DataAdapter/ARS308Adapter/leftFrontRadar/Subsystem1/OBJ_35 ==
  OBJ_01 : Inport
  Bus Creator : BusCreator  Inputs=2  OutDataTypeStr=Bus: FUS_UINT8_RESERVED_ST
      settings: InheritFromInputs=off
  Bus Creator1 : BusCreator  Inputs=17  OutDataTypeStr=Bus: FUS_RADAR_OBJ_ST  NonVirtualBus=on
      settings: InheritFromInputs=off
  Bus Selector1 : BusSelector  OutputSignals=RCS,VrelLat,VrelLong,DistLong,DistLat,ID,DynProp
  Constant{,1,8..10} (5 alike) : Constant  Value=0  OutDataTypeStr=uint8
  Constant{2..6} (5 alike) : Constant  Value=0  OutDataTypeStr=single
  Constant7 : Constant  OutDataTypeStr=uint8
  Data Type Conversion : DataTypeConversion  OutDataTypeStr=uint16
  Data Type Conversion1 : DataTypeConversion  OutDataTypeStr=uint8
  Switch : Switch  Criteria=u2 > Threshold  OutDataTypeStr=uint8
  <OBJ_01> : Outport
  wires:
  Constant1/1 -> Bus Creator/2
  Bus Creator1/1 -> <OBJ_01>/1
  Constant/1 -> Bus Creator/1
  OBJ_01/1 -> Bus Selector1/1
  Bus Creator/1 -> Bus Creator1/17
  Bus Selector1/1 -> Bus Creator1/1  "<RCS>"
  Constant2/1 -> Bus Creator1/2  "XPos_STD"
  Constant3/1 -> Bus Creator1/3  "YPos_STD"
  Constant4/1 -> Bus Creator1/4  "XVelRel_STD"
  Constant5/1 -> Bus Creator1/5  "XAccRel"
  Constant6/1 -> Bus Creator1/6  "ExstProb"
  Bus Selector1/2 -> Bus Creator1/7  "<VrelLat>"
  Bus Selector1/3 -> Bus Creator1/8  "<VrelLong>"
  Bus Selector1/4 -> Bus Creator1/9  "<DistLong>"
  Bus Selector1/5 -> Bus Creator1/10  "<DistLat>"
  Bus Selector1/6 -> Data Type Conversion/1  "<ID>"
  Data Type Conversion/1 -> Bus Creator1/11, Switch/2
  Constant8/1 -> Switch/3  "ValidFlag"
  Bus Selector1/7 -> Data Type Conversion1/1  "<DynProp>"
  Constant9/1 -> Bus Creator1/15  "Type"
  Constant10/1 -> Bus Creator1/16  "MeasFlag"
  Data Type Conversion1/1 -> Bus Creator1/14
  Constant7/1 -> Switch/1  "UpdateFlag"
  Switch/1 -> Bus Creator1/13, Bus Creator1/12

== system fusionAlg/FUSION /FUS_DataAdapter/ARS308Adapter/leftFrontRadar/Subsystem1/OBJ_36 ==
  OBJ_01 : Inport
  Bus Creator : BusCreator  Inputs=2  OutDataTypeStr=Bus: FUS_UINT8_RESERVED_ST
      settings: InheritFromInputs=off
  Bus Creator1 : BusCreator  Inputs=17  OutDataTypeStr=Bus: FUS_RADAR_OBJ_ST  NonVirtualBus=on
      settings: InheritFromInputs=off
  Bus Selector1 : BusSelector  OutputSignals=RCS,VrelLat,VrelLong,DistLong,DistLat,ID,DynProp
  Constant{,1,8..10} (5 alike) : Constant  Value=0  OutDataTypeStr=uint8
  Constant{2..6} (5 alike) : Constant  Value=0  OutDataTypeStr=single
  Constant7 : Constant  OutDataTypeStr=uint8
  Data Type Conversion : DataTypeConversion  OutDataTypeStr=uint16
  Data Type Conversion1 : DataTypeConversion  OutDataTypeStr=uint8
  Switch : Switch  Criteria=u2 > Threshold  OutDataTypeStr=uint8
  <OBJ_01> : Outport
  wires:
  Constant1/1 -> Bus Creator/2
  Bus Creator1/1 -> <OBJ_01>/1
  Constant/1 -> Bus Creator/1
  OBJ_01/1 -> Bus Selector1/1
  Bus Creator/1 -> Bus Creator1/17
  Bus Selector1/1 -> Bus Creator1/1  "<RCS>"
  Constant2/1 -> Bus Creator1/2  "XPos_STD"
  Constant3/1 -> Bus Creator1/3  "YPos_STD"
  Constant4/1 -> Bus Creator1/4  "XVelRel_STD"
  Constant5/1 -> Bus Creator1/5  "XAccRel"
  Constant6/1 -> Bus Creator1/6  "ExstProb"
  Bus Selector1/2 -> Bus Creator1/7  "<VrelLat>"
  Bus Selector1/3 -> Bus Creator1/8  "<VrelLong>"
  Bus Selector1/4 -> Bus Creator1/9  "<DistLong>"
  Bus Selector1/5 -> Bus Creator1/10  "<DistLat>"
  Bus Selector1/6 -> Data Type Conversion/1  "<ID>"
  Data Type Conversion/1 -> Bus Creator1/11, Switch/2
  Constant8/1 -> Switch/3  "ValidFlag"
  Bus Selector1/7 -> Data Type Conversion1/1  "<DynProp>"
  Constant9/1 -> Bus Creator1/15  "Type"
  Constant10/1 -> Bus Creator1/16  "MeasFlag"
  Data Type Conversion1/1 -> Bus Creator1/14
  Constant7/1 -> Switch/1  "UpdateFlag"
  Switch/1 -> Bus Creator1/13, Bus Creator1/12

== system fusionAlg/FUSION /FUS_DataAdapter/ARS308Adapter/leftFrontRadar/Subsystem1/OBJ_37 ==
  OBJ_01 : Inport
  Bus Creator : BusCreator  Inputs=2  OutDataTypeStr=Bus: FUS_UINT8_RESERVED_ST
      settings: InheritFromInputs=off
  Bus Creator1 : BusCreator  Inputs=17  OutDataTypeStr=Bus: FUS_RADAR_OBJ_ST  NonVirtualBus=on
      settings: InheritFromInputs=off
  Bus Selector1 : BusSelector  OutputSignals=RCS,VrelLat,VrelLong,DistLong,DistLat,ID,DynProp
  Constant{,1,8..10} (5 alike) : Constant  Value=0  OutDataTypeStr=uint8
  Constant{2..6} (5 alike) : Constant  Value=0  OutDataTypeStr=single
  Constant7 : Constant  OutDataTypeStr=uint8
  Data Type Conversion : DataTypeConversion  OutDataTypeStr=uint16
  Data Type Conversion1 : DataTypeConversion  OutDataTypeStr=uint8
  Switch : Switch  Criteria=u2 > Threshold  OutDataTypeStr=uint8
  <OBJ_01> : Outport
  wires:
  Constant1/1 -> Bus Creator/2
  Bus Creator1/1 -> <OBJ_01>/1
  Constant/1 -> Bus Creator/1
  OBJ_01/1 -> Bus Selector1/1
  Bus Creator/1 -> Bus Creator1/17
  Bus Selector1/1 -> Bus Creator1/1  "<RCS>"
  Constant2/1 -> Bus Creator1/2  "XPos_STD"
  Constant3/1 -> Bus Creator1/3  "YPos_STD"
  Constant4/1 -> Bus Creator1/4  "XVelRel_STD"
  Constant5/1 -> Bus Creator1/5  "XAccRel"
  Constant6/1 -> Bus Creator1/6  "ExstProb"
  Bus Selector1/2 -> Bus Creator1/7  "<VrelLat>"
  Bus Selector1/3 -> Bus Creator1/8  "<VrelLong>"
  Bus Selector1/4 -> Bus Creator1/9  "<DistLong>"
  Bus Selector1/5 -> Bus Creator1/10  "<DistLat>"
  Bus Selector1/6 -> Data Type Conversion/1  "<ID>"
  Data Type Conversion/1 -> Bus Creator1/11, Switch/2
  Constant8/1 -> Switch/3  "ValidFlag"
  Bus Selector1/7 -> Data Type Conversion1/1  "<DynProp>"
  Constant9/1 -> Bus Creator1/15  "Type"
  Constant10/1 -> Bus Creator1/16  "MeasFlag"
  Data Type Conversion1/1 -> Bus Creator1/14
  Constant7/1 -> Switch/1  "UpdateFlag"
  Switch/1 -> Bus Creator1/13, Bus Creator1/12

== system fusionAlg/FUSION /FUS_DataAdapter/ARS308Adapter/leftFrontRadar/Subsystem1/OBJ_38 ==
  OBJ_01 : Inport
  Bus Creator : BusCreator  Inputs=2  OutDataTypeStr=Bus: FUS_UINT8_RESERVED_ST
      settings: InheritFromInputs=off
  Bus Creator1 : BusCreator  Inputs=17  OutDataTypeStr=Bus: FUS_RADAR_OBJ_ST  NonVirtualBus=on
      settings: InheritFromInputs=off
  Bus Selector1 : BusSelector  OutputSignals=RCS,VrelLat,VrelLong,DistLong,DistLat,ID,DynProp
  Constant{,1,8..10} (5 alike) : Constant  Value=0  OutDataTypeStr=uint8
  Constant{2..6} (5 alike) : Constant  Value=0  OutDataTypeStr=single
  Constant7 : Constant  OutDataTypeStr=uint8
  Data Type Conversion : DataTypeConversion  OutDataTypeStr=uint16
  Data Type Conversion1 : DataTypeConversion  OutDataTypeStr=uint8
  Switch : Switch  Criteria=u2 > Threshold  OutDataTypeStr=uint8
  <OBJ_01> : Outport
  wires:
  Constant1/1 -> Bus Creator/2
  Bus Creator1/1 -> <OBJ_01>/1
  Constant/1 -> Bus Creator/1
  OBJ_01/1 -> Bus Selector1/1
  Bus Creator/1 -> Bus Creator1/17
  Bus Selector1/1 -> Bus Creator1/1  "<RCS>"
  Constant2/1 -> Bus Creator1/2  "XPos_STD"
  Constant3/1 -> Bus Creator1/3  "YPos_STD"
  Constant4/1 -> Bus Creator1/4  "XVelRel_STD"
  Constant5/1 -> Bus Creator1/5  "XAccRel"
  Constant6/1 -> Bus Creator1/6  "ExstProb"
  Bus Selector1/2 -> Bus Creator1/7  "<VrelLat>"
  Bus Selector1/3 -> Bus Creator1/8  "<VrelLong>"
  Bus Selector1/4 -> Bus Creator1/9  "<DistLong>"
  Bus Selector1/5 -> Bus Creator1/10  "<DistLat>"
  Bus Selector1/6 -> Data Type Conversion/1  "<ID>"
  Data Type Conversion/1 -> Bus Creator1/11, Switch/2
  Constant8/1 -> Switch/3  "ValidFlag"
  Bus Selector1/7 -> Data Type Conversion1/1  "<DynProp>"
  Constant9/1 -> Bus Creator1/15  "Type"
  Constant10/1 -> Bus Creator1/16  "MeasFlag"
  Data Type Conversion1/1 -> Bus Creator1/14
  Constant7/1 -> Switch/1  "UpdateFlag"
  Switch/1 -> Bus Creator1/13, Bus Creator1/12

== system fusionAlg/FUSION /FUS_DataAdapter/ARS308Adapter/leftFrontRadar/Subsystem1/OBJ_39 ==
  OBJ_01 : Inport
  Bus Creator : BusCreator  Inputs=2  OutDataTypeStr=Bus: FUS_UINT8_RESERVED_ST
      settings: InheritFromInputs=off
  Bus Creator1 : BusCreator  Inputs=17  OutDataTypeStr=Bus: FUS_RADAR_OBJ_ST  NonVirtualBus=on
      settings: InheritFromInputs=off
  Bus Selector1 : BusSelector  OutputSignals=RCS,VrelLat,VrelLong,DistLong,DistLat,ID,DynProp
  Constant{,1,8..10} (5 alike) : Constant  Value=0  OutDataTypeStr=uint8
  Constant{2..6} (5 alike) : Constant  Value=0  OutDataTypeStr=single
  Constant7 : Constant  OutDataTypeStr=uint8
  Data Type Conversion : DataTypeConversion  OutDataTypeStr=uint16
  Data Type Conversion1 : DataTypeConversion  OutDataTypeStr=uint8
  Switch : Switch  Criteria=u2 > Threshold  OutDataTypeStr=uint8
  <OBJ_01> : Outport
  wires:
  Constant1/1 -> Bus Creator/2
  Bus Creator1/1 -> <OBJ_01>/1
  Constant/1 -> Bus Creator/1
  OBJ_01/1 -> Bus Selector1/1
  Bus Creator/1 -> Bus Creator1/17
  Bus Selector1/1 -> Bus Creator1/1  "<RCS>"
  Constant2/1 -> Bus Creator1/2  "XPos_STD"
  Constant3/1 -> Bus Creator1/3  "YPos_STD"
  Constant4/1 -> Bus Creator1/4  "XVelRel_STD"
  Constant5/1 -> Bus Creator1/5  "XAccRel"
  Constant6/1 -> Bus Creator1/6  "ExstProb"
  Bus Selector1/2 -> Bus Creator1/7  "<VrelLat>"
  Bus Selector1/3 -> Bus Creator1/8  "<VrelLong>"
  Bus Selector1/4 -> Bus Creator1/9  "<DistLong>"
  Bus Selector1/5 -> Bus Creator1/10  "<DistLat>"
  Bus Selector1/6 -> Data Type Conversion/1  "<ID>"
  Data Type Conversion/1 -> Bus Creator1/11, Switch/2
  Constant8/1 -> Switch/3  "ValidFlag"
  Bus Selector1/7 -> Data Type Conversion1/1  "<DynProp>"
  Constant9/1 -> Bus Creator1/15  "Type"
  Constant10/1 -> Bus Creator1/16  "MeasFlag"
  Data Type Conversion1/1 -> Bus Creator1/14
  Constant7/1 -> Switch/1  "UpdateFlag"
  Switch/1 -> Bus Creator1/13, Bus Creator1/12

== system fusionAlg/FUSION /FUS_DataAdapter/ARS308Adapter/leftFrontRadar/Subsystem1/OBJ_4 ==
  OBJ_01 : Inport
  Bus Creator : BusCreator  Inputs=2  OutDataTypeStr=Bus: FUS_UINT8_RESERVED_ST
      settings: InheritFromInputs=off
  Bus Creator1 : BusCreator  Inputs=17  OutDataTypeStr=Bus: FUS_RADAR_OBJ_ST  NonVirtualBus=on
      settings: InheritFromInputs=off
  Bus Selector1 : BusSelector  OutputSignals=RCS,VrelLat,VrelLong,DistLong,DistLat,ID,DynProp
  Constant{,1,8..10} (5 alike) : Constant  Value=0  OutDataTypeStr=uint8
  Constant{2..6} (5 alike) : Constant  Value=0  OutDataTypeStr=single
  Constant7 : Constant  OutDataTypeStr=uint8
  Data Type Conversion : DataTypeConversion  OutDataTypeStr=uint16
  Data Type Conversion1 : DataTypeConversion  OutDataTypeStr=uint8
  Switch : Switch  Criteria=u2 > Threshold  OutDataTypeStr=uint8
  <OBJ_01> : Outport
  wires:
  Constant1/1 -> Bus Creator/2
  Bus Creator1/1 -> <OBJ_01>/1
  Constant/1 -> Bus Creator/1
  OBJ_01/1 -> Bus Selector1/1
  Bus Creator/1 -> Bus Creator1/17
  Bus Selector1/1 -> Bus Creator1/1  "<RCS>"
  Constant2/1 -> Bus Creator1/2  "XPos_STD"
  Constant3/1 -> Bus Creator1/3  "YPos_STD"
  Constant4/1 -> Bus Creator1/4  "XVelRel_STD"
  Constant5/1 -> Bus Creator1/5  "XAccRel"
  Constant6/1 -> Bus Creator1/6  "ExstProb"
  Bus Selector1/2 -> Bus Creator1/7  "<VrelLat>"
  Bus Selector1/3 -> Bus Creator1/8  "<VrelLong>"
  Bus Selector1/4 -> Bus Creator1/9  "<DistLong>"
  Bus Selector1/5 -> Bus Creator1/10  "<DistLat>"
  Bus Selector1/6 -> Data Type Conversion/1  "<ID>"
  Data Type Conversion/1 -> Bus Creator1/11, Switch/2
  Constant8/1 -> Switch/3  "ValidFlag"
  Bus Selector1/7 -> Data Type Conversion1/1  "<DynProp>"
  Constant9/1 -> Bus Creator1/15  "Type"
  Constant10/1 -> Bus Creator1/16  "MeasFlag"
  Data Type Conversion1/1 -> Bus Creator1/14
  Constant7/1 -> Switch/1  "UpdateFlag"
  Switch/1 -> Bus Creator1/13, Bus Creator1/12

== system fusionAlg/FUSION /FUS_DataAdapter/ARS308Adapter/leftFrontRadar/Subsystem1/OBJ_40 ==
  OBJ_01 : Inport
  Bus Creator : BusCreator  Inputs=2  OutDataTypeStr=Bus: FUS_UINT8_RESERVED_ST
      settings: InheritFromInputs=off
  Bus Creator1 : BusCreator  Inputs=17  OutDataTypeStr=Bus: FUS_RADAR_OBJ_ST  NonVirtualBus=on
      settings: InheritFromInputs=off
  Bus Selector1 : BusSelector  OutputSignals=RCS,VrelLat,VrelLong,DistLong,DistLat,ID,DynProp
  Constant{,1,8..10} (5 alike) : Constant  Value=0  OutDataTypeStr=uint8
  Constant{2..6} (5 alike) : Constant  Value=0  OutDataTypeStr=single
  Constant7 : Constant  OutDataTypeStr=uint8
  Data Type Conversion : DataTypeConversion  OutDataTypeStr=uint16
  Data Type Conversion1 : DataTypeConversion  OutDataTypeStr=uint8
  Switch : Switch  Criteria=u2 > Threshold  OutDataTypeStr=uint8
  <OBJ_01> : Outport
  wires:
  Constant1/1 -> Bus Creator/2
  Bus Creator1/1 -> <OBJ_01>/1
  Constant/1 -> Bus Creator/1
  OBJ_01/1 -> Bus Selector1/1
  Bus Creator/1 -> Bus Creator1/17
  Bus Selector1/1 -> Bus Creator1/1  "<RCS>"
  Constant2/1 -> Bus Creator1/2  "XPos_STD"
  Constant3/1 -> Bus Creator1/3  "YPos_STD"
  Constant4/1 -> Bus Creator1/4  "XVelRel_STD"
  Constant5/1 -> Bus Creator1/5  "XAccRel"
  Constant6/1 -> Bus Creator1/6  "ExstProb"
  Bus Selector1/2 -> Bus Creator1/7  "<VrelLat>"
  Bus Selector1/3 -> Bus Creator1/8  "<VrelLong>"
  Bus Selector1/4 -> Bus Creator1/9  "<DistLong>"
  Bus Selector1/5 -> Bus Creator1/10  "<DistLat>"
  Bus Selector1/6 -> Data Type Conversion/1  "<ID>"
  Data Type Conversion/1 -> Bus Creator1/11, Switch/2
  Constant8/1 -> Switch/3  "ValidFlag"
  Bus Selector1/7 -> Data Type Conversion1/1  "<DynProp>"
  Constant9/1 -> Bus Creator1/15  "Type"
  Constant10/1 -> Bus Creator1/16  "MeasFlag"
  Data Type Conversion1/1 -> Bus Creator1/14
  Constant7/1 -> Switch/1  "UpdateFlag"
  Switch/1 -> Bus Creator1/13, Bus Creator1/12

== system fusionAlg/FUSION /FUS_DataAdapter/ARS308Adapter/leftFrontRadar/Subsystem1/OBJ_5 ==
  OBJ_01 : Inport
  Bus Creator : BusCreator  Inputs=2  OutDataTypeStr=Bus: FUS_UINT8_RESERVED_ST
      settings: InheritFromInputs=off
  Bus Creator1 : BusCreator  Inputs=17  OutDataTypeStr=Bus: FUS_RADAR_OBJ_ST  NonVirtualBus=on
      settings: InheritFromInputs=off
  Bus Selector1 : BusSelector  OutputSignals=RCS,VrelLat,VrelLong,DistLong,DistLat,ID,DynProp
  Constant{,1,8..10} (5 alike) : Constant  Value=0  OutDataTypeStr=uint8
  Constant{2..6} (5 alike) : Constant  Value=0  OutDataTypeStr=single
  Constant7 : Constant  OutDataTypeStr=uint8
  Data Type Conversion : DataTypeConversion  OutDataTypeStr=uint16
  Data Type Conversion1 : DataTypeConversion  OutDataTypeStr=uint8
  Switch : Switch  Criteria=u2 > Threshold  OutDataTypeStr=uint8
  <OBJ_01> : Outport
  wires:
  Constant1/1 -> Bus Creator/2
  Bus Creator1/1 -> <OBJ_01>/1
  Constant/1 -> Bus Creator/1
  OBJ_01/1 -> Bus Selector1/1
  Bus Creator/1 -> Bus Creator1/17
  Bus Selector1/1 -> Bus Creator1/1  "<RCS>"
  Constant2/1 -> Bus Creator1/2  "XPos_STD"
  Constant3/1 -> Bus Creator1/3  "YPos_STD"
  Constant4/1 -> Bus Creator1/4  "XVelRel_STD"
  Constant5/1 -> Bus Creator1/5  "XAccRel"
  Constant6/1 -> Bus Creator1/6  "ExstProb"
  Bus Selector1/2 -> Bus Creator1/7  "<VrelLat>"
  Bus Selector1/3 -> Bus Creator1/8  "<VrelLong>"
  Bus Selector1/4 -> Bus Creator1/9  "<DistLong>"
  Bus Selector1/5 -> Bus Creator1/10  "<DistLat>"
  Bus Selector1/6 -> Data Type Conversion/1  "<ID>"
  Data Type Conversion/1 -> Bus Creator1/11, Switch/2
  Constant8/1 -> Switch/3  "ValidFlag"
  Bus Selector1/7 -> Data Type Conversion1/1  "<DynProp>"
  Constant9/1 -> Bus Creator1/15  "Type"
  Constant10/1 -> Bus Creator1/16  "MeasFlag"
  Data Type Conversion1/1 -> Bus Creator1/14
  Constant7/1 -> Switch/1  "UpdateFlag"
  Switch/1 -> Bus Creator1/13, Bus Creator1/12

== system fusionAlg/FUSION /FUS_DataAdapter/ARS308Adapter/leftFrontRadar/Subsystem1/OBJ_6 ==
  OBJ_01 : Inport
  Bus Creator : BusCreator  Inputs=2  OutDataTypeStr=Bus: FUS_UINT8_RESERVED_ST
      settings: InheritFromInputs=off
  Bus Creator1 : BusCreator  Inputs=17  OutDataTypeStr=Bus: FUS_RADAR_OBJ_ST  NonVirtualBus=on
      settings: InheritFromInputs=off
  Bus Selector1 : BusSelector  OutputSignals=RCS,VrelLat,VrelLong,DistLong,DistLat,ID,DynProp
  Constant{,1,8..10} (5 alike) : Constant  Value=0  OutDataTypeStr=uint8
  Constant{2..6} (5 alike) : Constant  Value=0  OutDataTypeStr=single
  Constant7 : Constant  OutDataTypeStr=uint8
  Data Type Conversion : DataTypeConversion  OutDataTypeStr=uint16
  Data Type Conversion1 : DataTypeConversion  OutDataTypeStr=uint8
  Switch : Switch  Criteria=u2 > Threshold  OutDataTypeStr=uint8
  <OBJ_01> : Outport
  wires:
  Constant1/1 -> Bus Creator/2
  Bus Creator1/1 -> <OBJ_01>/1
  Constant/1 -> Bus Creator/1
  OBJ_01/1 -> Bus Selector1/1
  Bus Creator/1 -> Bus Creator1/17
  Bus Selector1/1 -> Bus Creator1/1  "<RCS>"
  Constant2/1 -> Bus Creator1/2  "XPos_STD"
  Constant3/1 -> Bus Creator1/3  "YPos_STD"
  Constant4/1 -> Bus Creator1/4  "XVelRel_STD"
  Constant5/1 -> Bus Creator1/5  "XAccRel"
  Constant6/1 -> Bus Creator1/6  "ExstProb"
  Bus Selector1/2 -> Bus Creator1/7  "<VrelLat>"
  Bus Selector1/3 -> Bus Creator1/8  "<VrelLong>"
  Bus Selector1/4 -> Bus Creator1/9  "<DistLong>"
  Bus Selector1/5 -> Bus Creator1/10  "<DistLat>"
  Bus Selector1/6 -> Data Type Conversion/1  "<ID>"
  Data Type Conversion/1 -> Bus Creator1/11, Switch/2
  Constant8/1 -> Switch/3  "ValidFlag"
  Bus Selector1/7 -> Data Type Conversion1/1  "<DynProp>"
  Constant9/1 -> Bus Creator1/15  "Type"
  Constant10/1 -> Bus Creator1/16  "MeasFlag"
  Data Type Conversion1/1 -> Bus Creator1/14
  Constant7/1 -> Switch/1  "UpdateFlag"
  Switch/1 -> Bus Creator1/13, Bus Creator1/12

== system fusionAlg/FUSION /FUS_DataAdapter/ARS308Adapter/leftFrontRadar/Subsystem1/OBJ_7 ==
  OBJ_01 : Inport
  Bus Creator : BusCreator  Inputs=2  OutDataTypeStr=Bus: FUS_UINT8_RESERVED_ST
      settings: InheritFromInputs=off
  Bus Creator1 : BusCreator  Inputs=17  OutDataTypeStr=Bus: FUS_RADAR_OBJ_ST  NonVirtualBus=on
      settings: InheritFromInputs=off
  Bus Selector1 : BusSelector  OutputSignals=RCS,VrelLat,VrelLong,DistLong,DistLat,ID,DynProp
  Constant{,1,8..10} (5 alike) : Constant  Value=0  OutDataTypeStr=uint8
  Constant{2..6} (5 alike) : Constant  Value=0  OutDataTypeStr=single
  Constant7 : Constant  OutDataTypeStr=uint8
  Data Type Conversion : DataTypeConversion  OutDataTypeStr=uint16
  Data Type Conversion1 : DataTypeConversion  OutDataTypeStr=uint8
  Switch : Switch  Criteria=u2 > Threshold  OutDataTypeStr=uint8
  <OBJ_01> : Outport
  wires:
  Constant1/1 -> Bus Creator/2
  Bus Creator1/1 -> <OBJ_01>/1
  Constant/1 -> Bus Creator/1
  OBJ_01/1 -> Bus Selector1/1
  Bus Creator/1 -> Bus Creator1/17
  Bus Selector1/1 -> Bus Creator1/1  "<RCS>"
  Constant2/1 -> Bus Creator1/2  "XPos_STD"
  Constant3/1 -> Bus Creator1/3  "YPos_STD"
  Constant4/1 -> Bus Creator1/4  "XVelRel_STD"
  Constant5/1 -> Bus Creator1/5  "XAccRel"
  Constant6/1 -> Bus Creator1/6  "ExstProb"
  Bus Selector1/2 -> Bus Creator1/7  "<VrelLat>"
  Bus Selector1/3 -> Bus Creator1/8  "<VrelLong>"
  Bus Selector1/4 -> Bus Creator1/9  "<DistLong>"
  Bus Selector1/5 -> Bus Creator1/10  "<DistLat>"
  Bus Selector1/6 -> Data Type Conversion/1  "<ID>"
  Data Type Conversion/1 -> Bus Creator1/11, Switch/2
  Constant8/1 -> Switch/3  "ValidFlag"
  Bus Selector1/7 -> Data Type Conversion1/1  "<DynProp>"
  Constant9/1 -> Bus Creator1/15  "Type"
  Constant10/1 -> Bus Creator1/16  "MeasFlag"
  Data Type Conversion1/1 -> Bus Creator1/14
  Constant7/1 -> Switch/1  "UpdateFlag"
  Switch/1 -> Bus Creator1/13, Bus Creator1/12
